simulink model "scheme3"  (R2022b)
settings: Solver=VariableStepAuto  StartTime=0.0  StopTime=10  MaxStep=0.01  RelTol=1e-3
values from neighbouring files (symbols this model uses):
  A = [0 1 ... (first row only)    [task3.m]
  B = [0; 1]    [task3.m]
  K = Y*P^-1    [task3.m]
  x0 = [1; 1]    [task3.m]
settings Model: Creator=alyok  LastModifiedBy=alyok

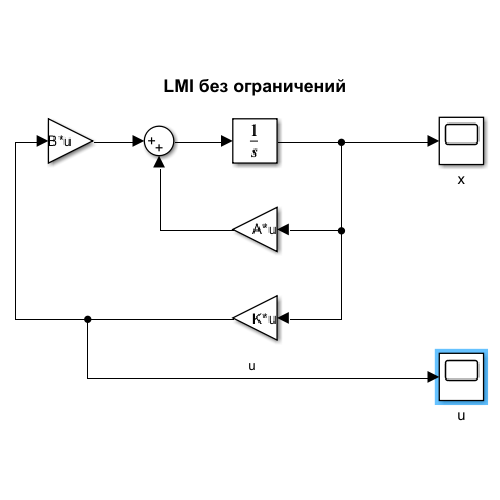
[thumbnail: Simulink's stored preview of the top-level diagram]
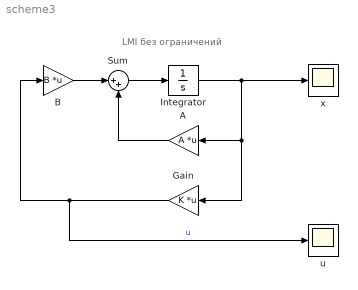
== system scheme3 ==
  note: LMI без ограничений
  A : Gain  Gain=A  Multiplication=Matrix(K*u)
  B : Gain  Gain=B  Multiplication=Matrix(K*u)
  Gain : Gain  Gain=K  Multiplication=Matrix(K*u)
  Integrator : Integrator  InitialCondition=x0
  Sum : Sum  Inputs=|++
  u : Scope
  x : Scope
  wires:
  Integrator/1 -> Gain/1, A/1, x/1
  Gain/1 -> u/1, B/1  "u"
  Sum/1 -> Integrator/1
  A/1 -> Sum/2
  B/1 -> Sum/1
